simulink model "designProject_Lead_Lag_cox"  (R2021a)
settings: Solver=VariableStepAuto  StartTime=0.0  StopTime=20  RelTol=1e-3
settings Model: Creator=Reaper124  LastModifiedBy=Reaper124

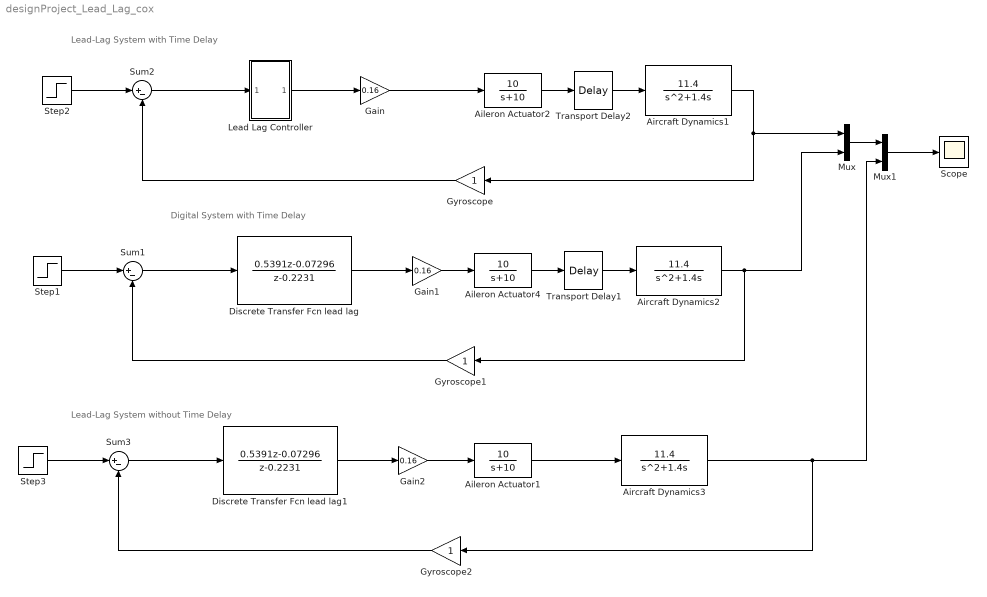
== system designProject_Lead_Lag_cox ==
  note: Lead-Lag System with Time Delay
  note: Digital System with Time Delay
  note: Lead-Lag System without Time Delay
  Aileron Actuator1 : TransferFcn  Numerator=[10]  Denominator=[1 10]
  Aileron Actuator2 : TransferFcn  Numerator=[10]  Denominator=[1 10]
  Aileron Actuator4 : TransferFcn  Numerator=[10]  Denominator=[1 10]
  Aircraft Dynamics1 : TransferFcn  Numerator=[11.4]  Denominator=[1 1.4 0]
  Aircraft Dynamics2 : TransferFcn  Numerator=[11.4]  Denominator=[1 1.4 0]
  Aircraft Dynamics3 : TransferFcn  Numerator=[11.4]  Denominator=[1 1.4 0]
  Discrete Transfer Fcn lead lag : DiscreteTransferFcn  Numerator=[0.5391 -0.07296]  Denominator=[1 -0.2231]  SampleTime=0.05
  Discrete Transfer Fcn lead lag1 : DiscreteTransferFcn  Numerator=[0.5391 -0.07296]  Denominator=[1 -0.2231]  SampleTime=0.05
  Gain : Gain  Gain=0.16
  Gain1 : Gain  Gain=0.16
  Gain2 : Gain  Gain=0.16
  Gyroscope : Gain
  Gyroscope1 : Gain
  Gyroscope2 : Gain
  Lead Lag Controller : Subsystem
  Mux : Mux  Inputs=2
  Mux1 : Mux  Inputs=2
  Scope : Scope
  Step1 : Step  SampleTime=0.05
  Step2 : Step  SampleTime=0
  Step3 : Step  SampleTime=0.05
  Sum1 : Sum  Inputs=|+-
  Sum2 : Sum  Inputs=|+-
  Sum3 : Sum  Inputs=|+-
  Transport Delay1 : TransportDelay  DelayTime=0.125
  Transport Delay2 : TransportDelay  DelayTime=0.125
  wires:
  Step2/1 -> Sum2/1
  Aileron Actuator2/1 -> Transport Delay2/1
  Transport Delay2/1 -> Aircraft Dynamics1/1
  Aircraft Dynamics1/1 -> Mux/1, Gyroscope/1
  Gyroscope/1 -> Sum2/2
  Gain/1 -> Aileron Actuator2/1
  Gyroscope1/1 -> Sum1/2
  Gain1/1 -> Aileron Actuator4/1
  Step1/1 -> Sum1/1
  Aileron Actuator4/1 -> Transport Delay1/1
  Aircraft Dynamics2/1 -> Gyroscope1/1, Mux/2
  Transport Delay1/1 -> Aircraft Dynamics2/1
  Sum2/1 -> Lead Lag Controller/1(In1)
  Lead Lag Controller/1(Out1) -> Gain/1
  Discrete Transfer Fcn lead lag/1 -> Gain1/1
  Sum1/1 -> Discrete Transfer Fcn lead lag/1
  Sum3/1 -> Discrete Transfer Fcn lead lag1/1
  Aircraft Dynamics3/1 -> Mux1/2, Gyroscope2/1
  Step3/1 -> Sum3/1
  Aileron Actuator1/1 -> Aircraft Dynamics3/1
  Discrete Transfer Fcn lead lag1/1 -> Gain2/1
  Gain2/1 -> Aileron Actuator1/1
  Gyroscope2/1 -> Sum3/2
  Mux/1 -> Mux1/1
  Mux1/1 -> Scope/1

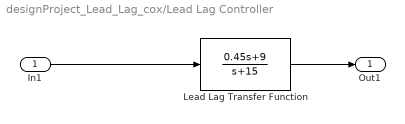
== system designProject_Lead_Lag_cox/Lead Lag Controller ==
  In1 : Inport
  Lead Lag Transfer Function : TransferFcn  Numerator=[0.45 9]  Denominator=[1 15]
  Out1 : Outport
  wires:
  In1/1 -> Lead Lag Transfer Function/1
  Lead Lag Transfer Function/1 -> Out1/1
